simulink model "ppr2"  (R2015b)
settings: Solver=VariableStepAuto  StartTime=0.0  StopTime=1e-5  RelTol=1e-3
libraries: dsparch4 x1, commsynccomp2 x1
settings Model: Creator=dimple  LastModifiedBy=dimple

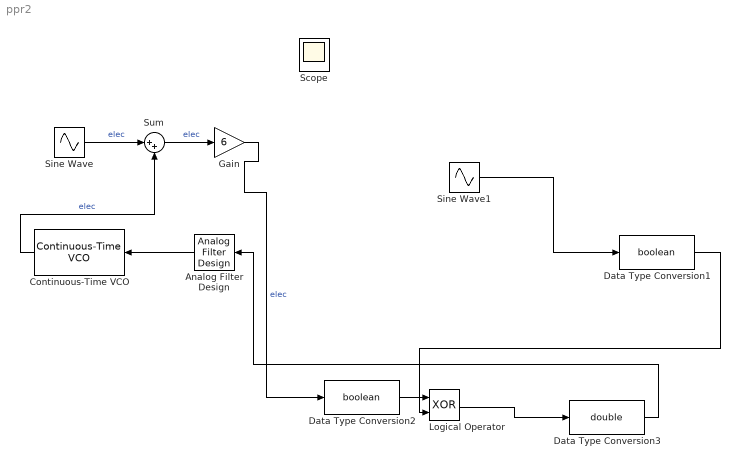
== system ppr2 ==
  Analog Filter Design : dsparch4/Analog Filter Design  method=Butterworth  filttype=Lowpass  N=5  Wlo=10e6  Whi=80  Rp=2  Rs=40
  Continuous-Time VCO : commsynccomp2/Continuous-Time VCO  Ac=10  Fc=1e5  Kc=1e6  Ph=0
  Data Type Conversion1 : DataTypeConversion  OutDataTypeStr=boolean
  Data Type Conversion2 : DataTypeConversion  OutDataTypeStr=boolean
  Data Type Conversion3 : DataTypeConversion  OutDataTypeStr=double
  Gain : Gain  Gain=6
  Logical Operator : Logic  Operator=XOR  AllPortsSameDT=off  OutDataTypeStr=fixdt(1,16)
  Scope : Scope  NumInputPorts=2
  Sine Wave : Sin  Amplitude=10  Frequency=1e6  SampleTime=0
  Sine Wave1 : Sin  Amplitude=10  Frequency=1e6  Phase=2  SampleTime=0
  Sum : Sum  Inputs=|++
  wires:
  Sine Wave/1 -> Sum/1  "elec"
  Analog Filter Design/1 -> Continuous-Time VCO/1
  Sum/1 -> Gain/1  "elec"
  Continuous-Time VCO/1 -> Sum/2  "elec"
  Gain/1 -> Data Type Conversion2/1  "elec"
  Data Type Conversion2/1 -> Logical Operator/1
  Sine Wave1/1 -> Data Type Conversion1/1
  Data Type Conversion1/1 -> Logical Operator/2
  Logical Operator/1 -> Data Type Conversion3/1
  Data Type Conversion3/1 -> Analog Filter Design/1
